simulink model "sampleSim"  (R2019a)
settings: Solver=VariableStepAuto  StartTime=0.0  StopTime=10.0  RelTol=1e-3
values from neighbouring files (symbols this model uses):
  b = 0.3/2    (= 0.15)    [dynamicControl.m]    (also in linearizedPlant.m; metaAlgorithm.m; metaAlgorithmAdvanced.m; returnLinearisedPlant.m = c(1))
  D = 2*b    (= 0.3)    [dynamicControl.m]    (also in linearizedPlant.m; metaAlgorithm.m; metaAlgorithmAdvanced.m; returnLinearisedPlant.m = c(2))
  J = 0.03    [dynamicControl.m]    (also in linearizedPlant.m; metaAlgorithm.m; metaAlgorithmAdvanced.m; returnLinearisedPlant.m = c(6))
  K = 1    [dynamicControl.m]    (also in linearizedPlant.m; metaAlgorithm.m; metaAlgorithmAdvanced.m; returnLinearisedPlant.m = c(7))
  m = 0.5    [dynamicControl.m]    (also in linearizedPlant.m; metaAlgorithm.m; metaAlgorithmAdvanced.m; returnLinearisedPlant.m = c(4))
  r = 0.05    [dynamicControl.m]    (also in linearizedPlant.m; metaAlgorithm.m; metaAlgorithmAdvanced.m; plantModel.m = constants(5))
  T = 0.01    [dynamicControl.m]    (also in linearizedPlant.m; metaAlgorithm.m; metaAlgorithmAdvanced.m; plantModel.m = constants(3))
settings Model: Creator=bhatt  LastModifiedBy=bhatt

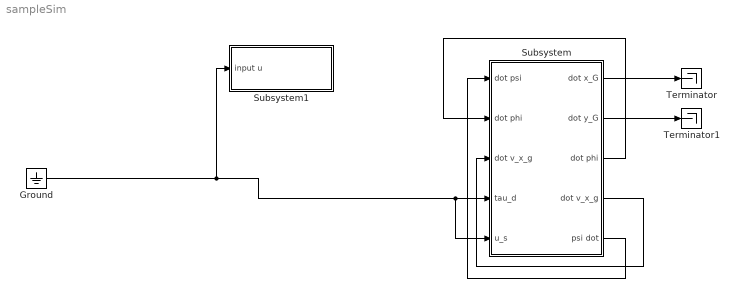
== system sampleSim ==
  Ground : Ground
  Subsystem : Subsystem
  Subsystem1 : Subsystem
  Terminator : Terminator
  Terminator1 : Terminator
  wires:
  Subsystem/5("psi dot ") -> Subsystem/1(dot psi)
  Subsystem/4("dot v_x_g ") -> Subsystem/3("dot v_x_g ")
  Subsystem/3(dot phi) -> Subsystem/2("dot phi ")
  Subsystem/1(dot x_G) -> Terminator/1
  Subsystem/2("dot y_G ") -> Terminator1/1
  Ground/1 -> Subsystem1/1("input u "), Subsystem/4(tau_d), Subsystem/5(u_s)

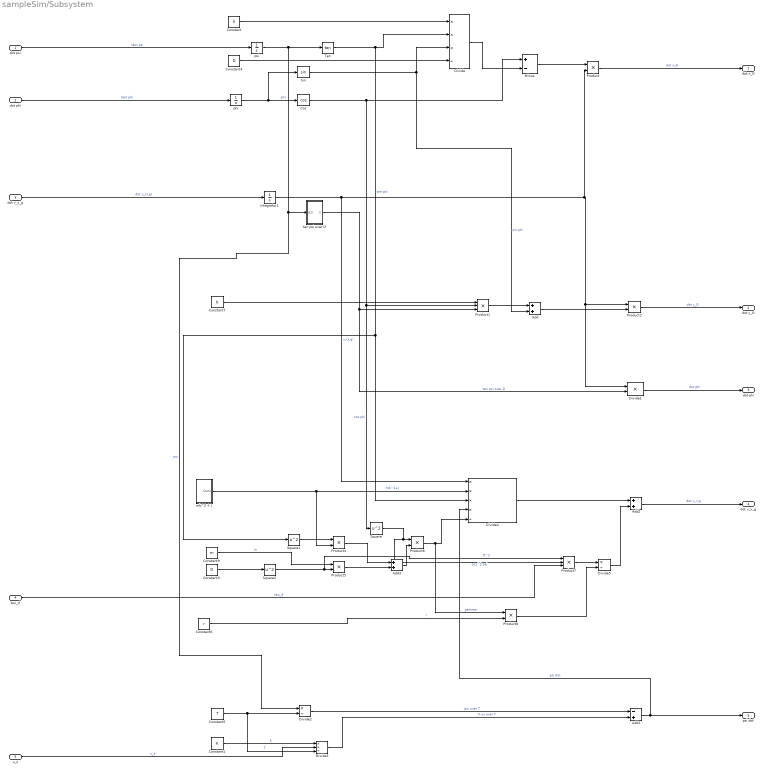
== system sampleSim/Subsystem ==
  dot psi : Inport
  "dot phi " : Inport  Port=2
  "dot v_x_g " : Inport  Port=3
  tau_d : Inport  Port=4
  u_s : Inport  Port=5
  Add : Sum
  Add1 : Sum  Inputs=-+
  Add2 : Sum
  Add3 : Sum
  Constant : Constant  Value=b
  Constant1 : Constant  Value=K
  Constant3 : Constant  Value=D
  Constant4 : Constant  Value=D
  Constant5 : Constant  Value=T
  Constant6 : Constant  Value=r
  Constant7 : Constant  Value=b
  Constant9 : Constant  Value=m
  Cos : Trigonometry  Operator=cos
  Divide : Product  Inputs=***/
  Divide1 : Product  Inputs=**
  Divide2 : Product  Inputs=*/
  Divide3 : Product  Inputs=**/
  Divide4 : Product  Inputs=****/
  Divide5 : Product  Inputs=*/
  Integrator1 : Integrator
  Minus : Sum  Inputs=+-
  Product{,2,4..6,8} (6 alike) : Product
  Product1 : Product  Inputs=3
  Product7 : Product  Inputs=3
  Sin : Trigonometry
  Square : Math  Operator=square  SaturateOnIntegerOverflow=on
  Square1 : Math  Operator=square  SaturateOnIntegerOverflow=on
  Square2 : Math  Operator=square  SaturateOnIntegerOverflow=on
  Tan : Trigonometry  Operator=tan
  mb^2 + J : Subsystem
  phi : Integrator
  psi : Integrator
  "tan psi over D " : Subsystem
  dot x_G : Outport
  "dot y_G " : Outport  Port=2
  dot phi : Outport  Port=3
  "dot v_x_g " : Outport  Port=4
  "psi dot " : Outport  Port=5
  wires:
  Constant5/1 -> Divide3/3, Divide2/2  "T"
  Constant3/1 -> Square2/1
  "tan psi over D "/1(Out1) -> Divide1/2, Product1/3  "tan psi over D"
  Divide4/1 -> Add2/1
  Constant7/1 -> Product1/1
  Divide1/1 -> dot phi/1  "dot phi"
  "dot phi "/1 -> phi/1  "\\dot phi"
  Constant1/1 -> Divide3/1  "K"
  mb^2 + J/1(Out1) -> Divide4/2, Product4/2  "mb^2+J"
  Add2/1 -> "dot v_x_g "/1  "dot v_x,g"
  Add/1 -> Product2/2
  Minus/1 -> Product/1
  Product5/1 -> Add3/2
  Divide/1 -> Minus/2
  Tan/1 -> Divide4/3, Square1/1, Divide/2  "tan psi"
  u_s/1 -> Divide3/2  "u_s"
  Square1/1 -> Product4/1
  Constant9/1 -> Product5/1  "m"
  Cos/1 -> Square/1, Product1/2, Minus/1  "cos phi"
  psi/1 -> Divide2/1, "tan psi over D "/1(psi), Tan/1  "psi"
  Square2/1 -> Product7/1, Product5/2  "D^2"
  dot psi/1 -> psi/1  "\\dot psi"
  Product/1 -> dot x_G/1  "dot x_G"
  Product1/1 -> Add/1
  Product8/1 -> Divide5/2
  tau_d/1 -> Product7/3  "tau_d"
  "dot v_x_g "/1 -> Integrator1/1  "dot v_(x,g)"
  Sin/1 -> Add/2, Divide/3  "sin phi"
  Constant/1 -> Divide/1
  Divide5/1 -> Add2/2
  Constant4/1 -> Divide/4
  Add1/1 -> "psi dot "/1, Divide4/4  "psi dot"
  Product4/1 -> Add3/1
  Product2/1 -> "dot y_G "/1  "dot y_G"
  Add3/1 -> Product6/2
  Product6/1 -> Product8/1, Divide4/5  "gamma"
  Divide3/1 -> Add1/2  "K us over T"
  Divide2/1 -> Add1/1  "psi over T"
  phi/1 -> Sin/1, Cos/1  "phi"
  Integrator1/1 -> Divide1/1, Product2/1, Product/2, Divide4/1  "v_(x,g)"
  Product7/1 -> Divide5/1
  Constant6/1 -> Product8/2  "r"
  Square/1 -> Product7/2, Product6/1  "cos^2 psi"

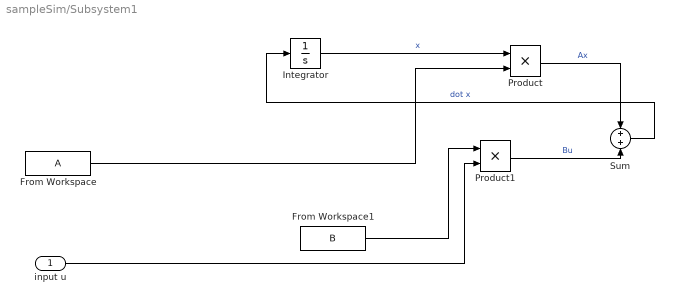
== system sampleSim/Subsystem1 ==
  "input u " : Inport
  From Workspace : FromWorkspace  VariableName=A  SampleTime=0
  From Workspace1 : FromWorkspace  VariableName=B  SampleTime=0
  Integrator : Integrator
  Product : Product
  Product1 : Product
  Sum : Sum  Inputs=2
  wires:
  Integrator/1 -> Product/1  "x"
  From Workspace/1 -> Product/2
  From Workspace1/1 -> Product1/1
  "input u "/1 -> Product1/2
  Product/1 -> Sum/1  "Ax"
  Product1/1 -> Sum/2  "Bu"
  Sum/1 -> Integrator/1  "dot x"

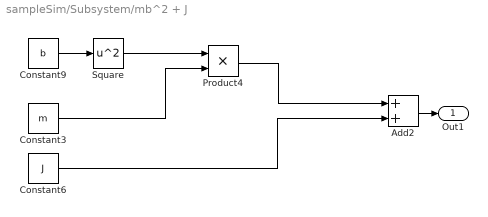
== system sampleSim/Subsystem/mb^2 + J ==
  Add2 : Sum
  Constant3 : Constant  Value=m
  Constant6 : Constant  Value=J
  Constant9 : Constant  Value=b
  Product4 : Product
  Square : Math  Operator=square  SaturateOnIntegerOverflow=on
  Out1 : Outport
  wires:
  Square/1 -> Product4/1
  Product4/1 -> Add2/1
  Add2/1 -> Out1/1
  Constant9/1 -> Square/1
  Constant3/1 -> Product4/2
  Constant6/1 -> Add2/2

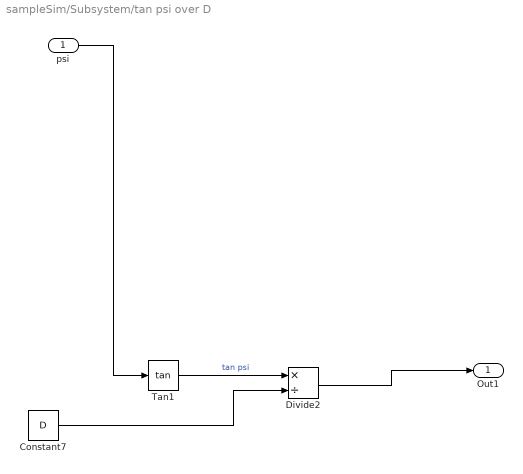
== system sampleSim/Subsystem/tan psi over D  ==
  psi : Inport
  Constant7 : Constant  Value=D
  Divide2 : Product  Inputs=*/
  Tan1 : Trigonometry  Operator=tan
  Out1 : Outport
  wires:
  Constant7/1 -> Divide2/2
  Tan1/1 -> Divide2/1  "tan psi"
  psi/1 -> Tan1/1
  Divide2/1 -> Out1/1
